simulink model "flyback"  (R2017b)
settings: Solver=FixedStepAuto  StartTime=0.0  StopTime=0.005  FixedStep=1e-8  MaxStep=1e-4  RelTol=1e-3
libraries: powerlib x16, powerlib_meascontrol x4
settings Model: Creator=tunay  LastModifiedBy=user
settings CodeAppCC: StateflowObjectComments=on
settings SimscapeCC: SimscapeNormalizeSystem=off

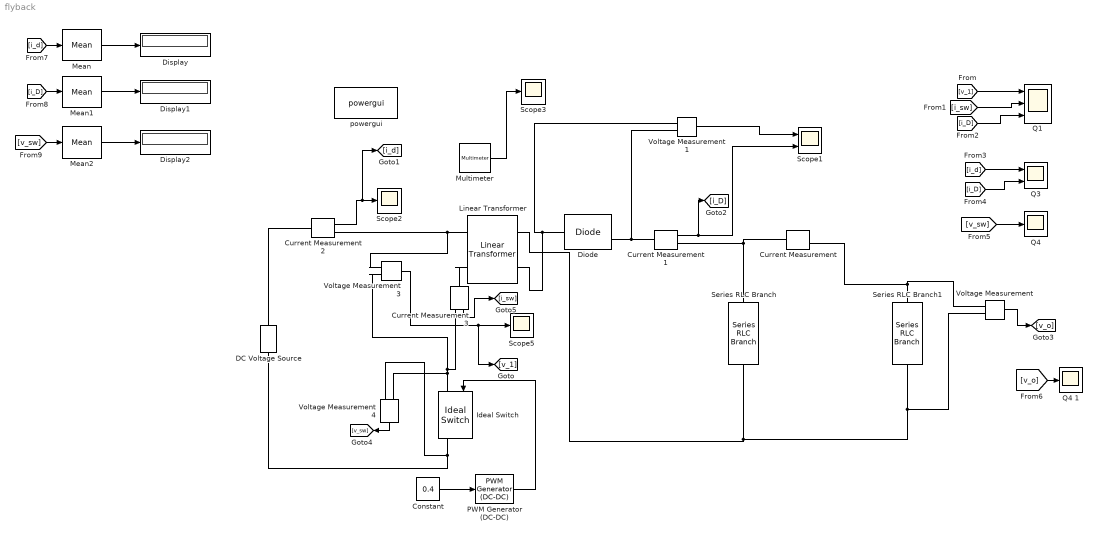
== system flyback ==
  Constant : Constant  Value=0.4
  Current Measurement{,1..3} (4 alike) : powerlib/Measurements/Current Measurement  PhasorSimulation=off  OutputType=Complex  PSBequivalent=0
  DC Voltage Source : powerlib/Electrical Sources/DC Voltage Source  Amplitude=310  Measurements=None
  Diode : powerlib/Power Electronics/Diode  Ron=0.001  Lon=0  Vf=0.8  IC=0  UseSnubber=0  Rs=500  Cs=250e-9  Measurements=on
  Display : Display
  Display1 : Display
  Display2 : Display
  Ideal Switch : powerlib/Power Electronics/Ideal Switch  Ron=0.6e-3  Lon=0  IC=0  Rs=1e5  Cs=inf  Measurements=on
  Linear Transformer : powerlib/Elements/Linear Transformer  UNITS=SI  NominalPower="[ 150  100e3 ]"  winding1=[124 0 0]  winding2=[10.33 0 0]  ThreeWindings=off  winding3=[3.15e+05 1.323e+06 105.28]  RmLm=[inf 40e-6]  Measurements=Winding currents  DataType=on
  Mean : powerlib_meascontrol/Measurements/Mean  Freq=100e3  Vinit=0  Ts=0
  Mean1 : powerlib_meascontrol/Measurements/Mean  Freq=100e3  Vinit=0  Ts=0
  Mean2 : powerlib_meascontrol/Measurements/Mean  Freq=100e3  Vinit=0  Ts=0
  Multimeter : powerlib/Measurements/Multimeter  PhasorSimulation=off  OutputType=Complex  sel=1  L=2  Gain=1  yselected={'Iw1: Linear Transformer'};  PSBOutputType=1  PSBequivalent=0  AxesSetting=[0,0.1,-100,100]  Display=0  SavedBlockNames=-11
  PWM Generator (DC-DC) : powerlib_meascontrol/Pulse & Signal Generators/PWM Generator (DC-DC)  Fsw=100e3  Ts=1e-8
  "Q1 " : Scope  NumInputPorts=3
  "Q3 " : Scope  NumInputPorts=2
  "Q4 " : Scope
  Q4 1 : Scope
  Scope1 : Scope  NumInputPorts=2
  Scope2 : Scope
  Scope3 : Scope
  Scope5 : Scope
  Series RLC Branch : powerlib/Elements/Series RLC Branch  LConnTagsString=__new0  RConnTagsString=__new0  BranchType=C  Resistance=1  Inductance=1e-3  SetiL0=off  InitialCurrent=0  Capacitance=200e-6  Setx0=off  InitialVoltage=15  Measurements=None
  Series RLC Branch1 : powerlib/Elements/Series RLC Branch  LConnTagsString=__new0  RConnTagsString=__new0  BranchType=R  Resistance=2  Inductance=1e-3  SetiL0=off  InitialCurrent=0  Capacitance=1e-6  Setx0=off  InitialVoltage=0  Measurements=None
  Voltage Measurement{,1,3..4} (4 alike) : powerlib/Measurements/Voltage Measurement  PhasorSimulation=off  OutputType=Complex  PSBequivalent=0
  powergui : powerlib/powergui  Priority=1  SimulationMode=Discrete  SampleTime=1e-8  frequency=60  Iterations=50  frequencyindice=0  Pbase=100e6  ErrMax=1e-4  UnitsV=kV  UnitsW=MW  buscounter=0  FunctionMessages=off  echomessages=off  EnableUseOfTLC=off  CurrentSourceSwitches=off  DisableSnubberDevices=off  DisableRonSwitches=off  DisableVfSwitches=off  DisplayEquations=off  SolverType=Tustin/Backward Euler (TBE)  Interpol=off  ExternalGateDelay=off  methode=off  Ts=100  x0status=blocks  SPID=off  SwTol=0  HookPort=off  RestoreLinks=warning  ResistiveCurrentMeasurement=off  Frange=[0:2:500]  Ylog=off  Xlog=on  ShowGrid=off  save=off  variable=ZData  structure=0  ZoomFFT=off  StartTime=0.0  cycles=1  DisplayStyle=1  fundamental=60  FreqAxis=off  MaxFrequency=1000  frequencyindicesteady=1  RmsSteady=1  display=off
  wires:
  PWM Generator (DC-DC)/1 -> Ideal Switch/1
  Constant/1 -> PWM Generator (DC-DC)/1
  Voltage Measurement/1 -> [v_o]
  Voltage Measurement1/1 -> Scope1/1
  Current Measurement1/1 -> [i_D], Scope1/2
  Current Measurement2/1 -> [i_d], Scope2/1
  Multimeter/1 -> Scope3/1
  Voltage Measurement3/1 -> [v_1], Scope5/1
  Voltage Measurement4/1 -> [v_sw]
  [v_1] -> "Q1 "/1
  [i_D] -> "Q1 "/3
  [i_sw] -> "Q1 "/2
  [i_d] -> "Q3 "/1
  [i_D] -> "Q3 "/2
  [v_sw] -> "Q4 "/1
  [v_o] -> Q4 1/1
  Current Measurement3/1 -> [i_sw]
  [i_d] -> Mean/1
  [i_D] -> Mean1/1
  Mean/1 -> Display/1
  Mean1/1 -> Display1/1
  Mean2/1 -> Display2/1
  [v_sw] -> Mean2/1
  connections:
  DC Voltage Source/LConn1 -- Voltage Measurement4/LConn2 -- Ideal Switch/RConn1
  Voltage Measurement1/LConn1 -- Diode/LConn1 -- Linear Transformer/RConn2
  Series RLC Branch/RConn1 -- Linear Transformer/RConn1 -- Voltage Measurement/LConn2 -- Series RLC Branch1/RConn1
  Voltage Measurement/LConn1 -- Current Measurement/RConn1 -- Series RLC Branch1/LConn1
  Series RLC Branch/LConn1 -- Current Measurement1/RConn1 -- Current Measurement/LConn1
  Current Measurement1/LConn1 -- Voltage Measurement1/LConn2 -- Diode/RConn1
  Voltage Measurement3/LConn2 -- Current Measurement3/RConn1 -- Voltage Measurement4/LConn1 -- Ideal Switch/LConn1
  DC Voltage Source/RConn1 -- Current Measurement2/LConn1
  Current Measurement2/RConn1 -- Linear Transformer/LConn1 -- Voltage Measurement3/LConn1
  Linear Transformer/LConn2 -- Current Measurement3/LConn1
